simulink model "Exercitiul6"  (R2016a)
settings: Solver=VariableStepDiscrete  StartTime=0.0  StopTime=100  RelTol=1e-3
undefined symbols (not defined in the file): m, n
settings Model: Creator=Cristina  LastModifiedBy=Cristina

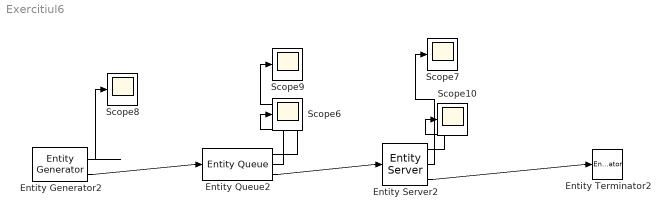
== system Exercitiul6 ==
  Entity Generator2 : EntityGenerator  OutputPortMessageModes=n,m  TimeSource=MATLAB action  IntergenerationTimeAction=dt = exprnd(0.2);  AttributeName=ServiceTime  NumberEntitiesDeparted=on  EntityType=Structured  EntityTypeName=Entity
      settings: OutputPortMap=o0,o3
  Entity Queue2 : EntityQueue  InputPortMessageModes=m  OutputPortMessageModes=n,n,m  NumberEntitiesDeparted=on  NumberEntitiesInBlock=on
      settings: OutputPortMap=o0,o1,o5
  Entity Server2 : EntityServer  InputPortMessageModes=m  OutputPortMessageModes=n,n,m  ServiceTimeSource=Attribute  ServiceTimeValue=1  ServiceTimeAction=dt = (1.2-0.8) * rand + 0.8  NumberEntitiesDeparted=on  NumberEntitiesInBlock=on
      settings: OutputPortMap=o0,o1,o9
  Entity Terminator2 : EntityTerminator  InputPortMessageModes=m
  Scope{6..10} (5 alike) : Scope
  wires:
  Entity Generator2/2 -> Entity Queue2/1
  Entity Queue2/3 -> Entity Server2/1
  Entity Server2/3 -> Entity Terminator2/1
  Entity Generator2/1 -> Scope8/1
  Entity Server2/1 -> Scope10/1
  Entity Queue2/2 -> Scope9/1
  Entity Queue2/1 -> Scope6/1
  Entity Server2/2 -> Scope7/1
